simulink model "SPWM copy"  (R2023b)
settings: Solver=VariableStepAuto  StartTime=0.0  StopTime=0.1  RelTol=1e-3
libraries: spsMosfetLib x6, spsSeriesRLCBranchLib x3, spsVoltageMeasurementLib x2, spsDCVoltageSourceLib x1, simulink x1, sps_lib x1
settings Model: Creator=saranshdhingra  LastModifiedBy=saranshdhingra
settings DataIOCC: SaveOutput=off  SaveState=on  SignalLogging=off  DSMLogging=off  ReturnWorkspaceOutputs=off

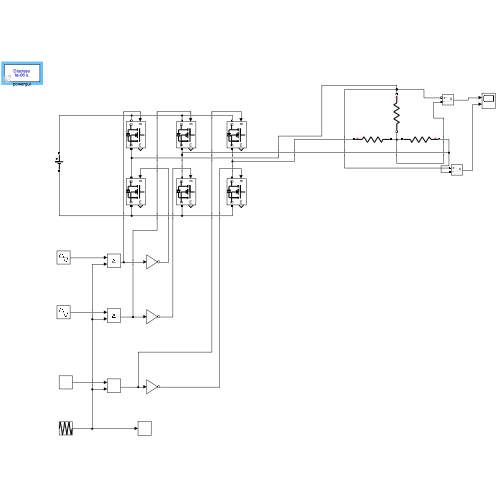
[thumbnail: Simulink's stored preview of the top-level diagram]
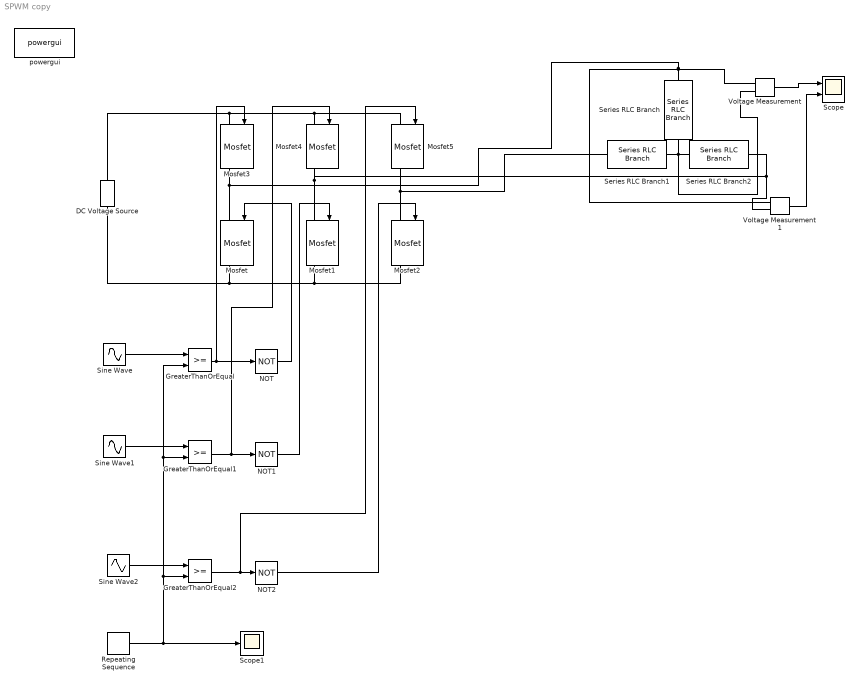
== system SPWM copy ==
  DC Voltage Source : spsDCVoltageSourceLib/DC Voltage Source  Amplitude=600  Measurements=Voltage
  GreaterThanOrEqual : RelationalOperator  OutDataTypeStr=boolean  RndMeth=Simplest  InputSameDT=off
  GreaterThanOrEqual1 : RelationalOperator  OutDataTypeStr=boolean  RndMeth=Simplest  InputSameDT=off
  GreaterThanOrEqual2 : RelationalOperator  OutDataTypeStr=boolean  RndMeth=Simplest  InputSameDT=off
  Mosfet{,1..5} (6 alike) : spsMosfetLib/Mosfet  Ron=0.1  Lon=0  Rd=0.01  Vfd=0  IC=0  Rs=1e5  Cs=inf  Measurements=on
  NOT : Logic  Operator=NOT  IconShape=distinctive  AllPortsSameDT=off  OutDataTypeStr=boolean
  NOT1 : Logic  Operator=NOT  IconShape=distinctive  AllPortsSameDT=off  OutDataTypeStr=boolean
  NOT2 : Logic  Operator=NOT  IconShape=distinctive  AllPortsSameDT=off  OutDataTypeStr=boolean
  Repeating Sequence : simulink/Sources/Repeating Sequence  rep_seq_t=[0 0.25 0.5 0.75 1] / 10000  rep_seq_y=[0 1 0 -1 0]
  Scope : Scope  NumInputPorts=2
  Scope1 : Scope
  Series RLC Branch : spsSeriesRLCBranchLib/Series RLC Branch  LConnTagsString=__new0  RConnTagsString=__new0  BranchType=R  Resistance=40  Inductance=0  SetiL0=off  InitialCurrent=0  Capacitance=0  Setx0=off  InitialVoltage=0  Measurements=None
  Series RLC Branch1 : spsSeriesRLCBranchLib/Series RLC Branch  LConnTagsString=__new0  RConnTagsString=__new0  BranchType=R  Resistance=40  Inductance=0  SetiL0=off  InitialCurrent=0  Capacitance=0  Setx0=off  InitialVoltage=0  Measurements=None
  Series RLC Branch2 : spsSeriesRLCBranchLib/Series RLC Branch  LConnTagsString=__new0  RConnTagsString=__new0  BranchType=R  Resistance=40  Inductance=0  SetiL0=off  InitialCurrent=0  Capacitance=0  Setx0=off  InitialVoltage=0  Measurements=None
  Sine Wave : Sin  Amplitude=230 / 300  Frequency=100*pi  SampleTime=0
  Sine Wave1 : Sin  Amplitude=230 / 300  Frequency=100 * pi  Phase=2*pi / 3  SampleTime=0
  Sine Wave2 : Sin  Amplitude=230 / 300  Frequency=100 * pi  Phase=4* pi / 3  SampleTime=0
  Voltage Measurement : spsVoltageMeasurementLib/Voltage Measurement  PhasorSimulation=off  OutputType=Complex  PSBequivalent=0
  Voltage Measurement1 : spsVoltageMeasurementLib/Voltage Measurement  PhasorSimulation=off  OutputType=Complex  PSBequivalent=0
  powergui : sps_lib/powergui  Priority=1  SimulationMode=Discrete  SampleTime=1e-6  frequency=60  Iterations=50  frequencyindice=0  Pbase=100e6  ErrMax=1e-4  UnitsV=kV  UnitsW=MW  buscounter=0  FunctionMessages=off  echomessages=off  EnableUseOfTLC=off  CurrentSourceSwitches=off  DisableSnubberDevices=off  DisableRonSwitches=off  DisableVfSwitches=off  DisplayEquations=off  AutomaticDiscreteSolvers=off  SolverType=Tustin/Backward Euler (TBE)  Interpol=off  ExternalGateDelay=off  methode=off  Ts=100  x0status=blocks  SPID=on  SwTol=0  HookPort=off  NonlinearTolerance=1e-4  nMaxIteration=100  ContinueOnMaxIteration=off  RestoreLinks=warning  ResistiveCurrentMeasurement=off  Frange=[0:2:500]  Ylog=off  Xlog=on  ShowGrid=off  save=off  variable=ZData  structure=0  ZoomFFT=off  StartTime=0.0  cycles=1  DisplayStyle=1  fundamental=60  FreqAxis=off  MaxFrequency=1000  frequencyindicesteady=1  RmsSteady=1  display=off
  wires:
  Sine Wave/1 -> GreaterThanOrEqual/1
  Sine Wave1/1 -> GreaterThanOrEqual1/1
  Sine Wave2/1 -> GreaterThanOrEqual2/1
  Repeating Sequence/1 -> Scope1/1, GreaterThanOrEqual1/2, GreaterThanOrEqual/2, GreaterThanOrEqual2/2
  GreaterThanOrEqual2/1 -> Mosfet5/1, NOT2/1
  GreaterThanOrEqual1/1 -> Mosfet4/1, NOT1/1
  GreaterThanOrEqual/1 -> NOT/1, Mosfet3/1
  NOT/1 -> Mosfet/1
  NOT1/1 -> Mosfet1/1
  NOT2/1 -> Mosfet2/1
  Voltage Measurement/1 -> Scope/1
  Voltage Measurement1/1 -> Scope/2
  connections:
  Mosfet3/LConn1 -- DC Voltage Source/RConn1 -- Mosfet5/LConn1 -- Mosfet4/LConn1
  Mosfet/RConn1 -- DC Voltage Source/LConn1 -- Mosfet2/RConn1 -- Mosfet1/RConn1
  Mosfet/LConn1 -- Voltage Measurement/LConn1 -- Voltage Measurement1/LConn1 -- Series RLC Branch/LConn1 -- Mosfet3/RConn1
  Mosfet1/LConn1 -- Series RLC Branch2/LConn1 -- Voltage Measurement1/LConn2 -- Mosfet4/RConn1
  Mosfet2/LConn1 -- Series RLC Branch1/LConn1 -- Mosfet5/RConn1
  Series RLC Branch2/RConn1 -- Voltage Measurement/LConn2 -- Series RLC Branch/RConn1 -- Series RLC Branch1/RConn1
